simulink model "Horticulture_Simulation_2"  (R2025a)
settings: Solver=ode45  StartTime=0.0  StopTime=100000  RelTol=1e-3
libraries: simulink x9, slpidlib x2
settings Model: Creator=VICTUS  LastModifiedBy=VICTUS

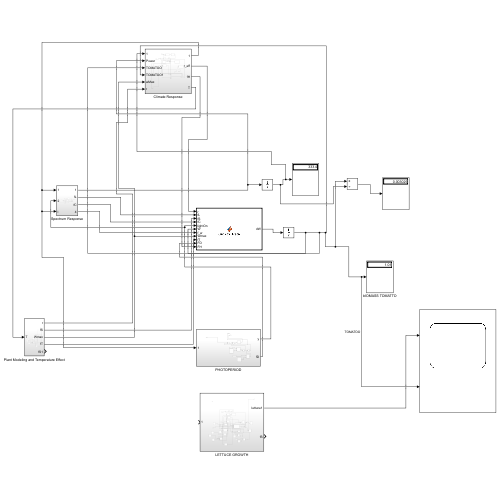
[thumbnail: Simulink's stored preview of the top-level diagram]
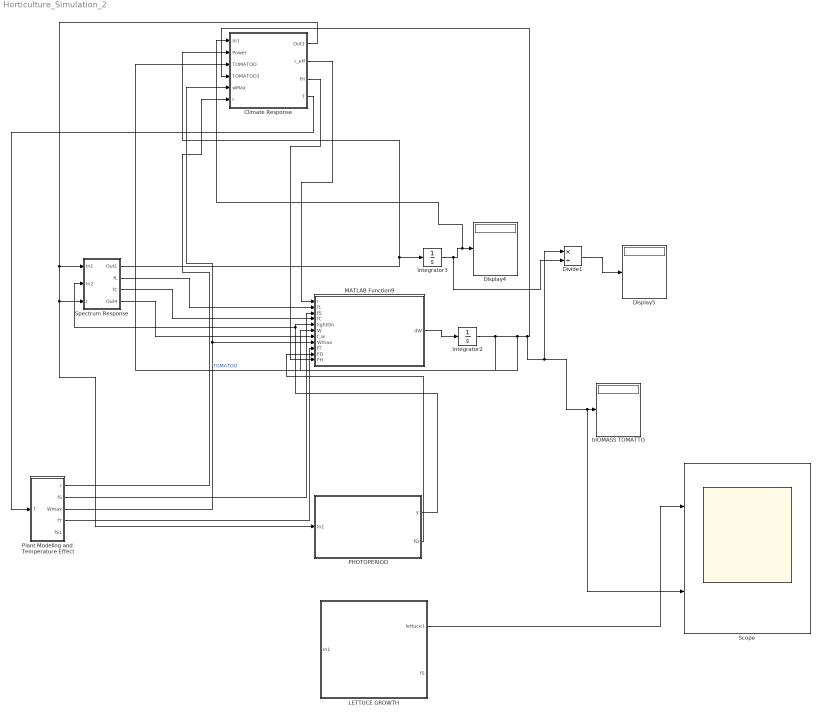
== system Horticulture_Simulation_2 ==
  Climate Response : Subsystem
  Display4 : Display
  Display5 : Display
  Divide1 : Product  Inputs=*/
  Integrator2 : Integrator  InitialCondition=1
  Integrator3 : Integrator
  LETTUCE GROWTH : Subsystem
  MATLAB Function9 : MATLAB Function  TreatAsAtomicUnit=on
  PHOTOPERIOD : Subsystem
  Plant Modeling and Temperature Effect : Subsystem
  Scope : Scope  NumInputPorts=2
      settings: ActiveDisplayYMinimum=0.99710090280302532  ActiveDisplayYMaximum=1.0260918747727719
  Spectrum Response : Subsystem
  bIOMASS TOMATTO : Display
  wires:
  Integrator2/1 -> Climate Response/3(TOMATOO), Climate Response/4(TOMATOO1), Divide1/1, Scope/2, bIOMASS TOMATTO/1, MATLAB Function9/6(W)  "TOMATOO"
  Divide1/1 -> Display5/1
  MATLAB Function9/1(dW) -> Integrator2/1
  Integrator3/1 -> Divide1/2, Climate Response/1(In1), Display4/1
  PHOTOPERIOD/1(y) -> Spectrum Response/2(In2), MATLAB Function9/5(lightOn)
  PHOTOPERIOD/2(fD) -> MATLAB Function9/10(FD)
  Plant Modeling and Temperature Effect/3(Wmax) -> Climate Response/5(wMax), MATLAB Function9/8(Wmax)
  Plant Modeling and Temperature Effect/2(fS) -> MATLAB Function9/3(fS)
  Plant Modeling and Temperature Effect/4(fT) -> MATLAB Function9/9(fT)
  Climate Response/1(Out1) -> PHOTOPERIOD/1(In1), Spectrum Response/3(I), Spectrum Response/1(In1)
  Plant Modeling and Temperature Effect/1(r) -> Climate Response/6(r)
  Climate Response/2(r_eff) -> MATLAB Function9/1(r)
  Climate Response/3(fH) -> MATLAB Function9/11(FH)
  Climate Response/4(T) -> Plant Modeling and Temperature Effect/1(T)
  Spectrum Response/1(Out1) -> Climate Response/2(Power), Integrator3/1
  Spectrum Response/2(fL) -> MATLAB Function9/2(fL)
  Spectrum Response/3(fC) -> MATLAB Function9/4(fC)
  Spectrum Response/4(Out4) -> MATLAB Function9/7(f_w)
  LETTUCE GROWTH/1(lettuce1) -> Scope/1

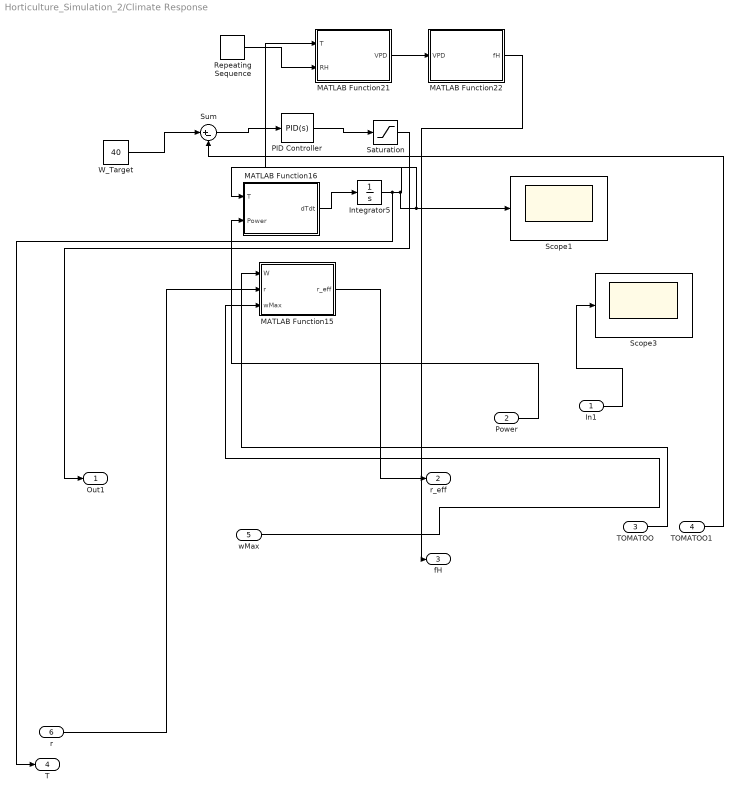
== system Horticulture_Simulation_2/Climate Response ==
  In1 : Inport
  Power : Inport  Port=2
  TOMATOO : Inport  Port=3
  TOMATOO1 : Inport  Port=4
  wMax : Inport  Port=5
  r : Inport  Port=6
  Integrator5 : Integrator  InitialCondition=22
  MATLAB Function15 : MATLAB Function  TreatAsAtomicUnit=on
  MATLAB Function16 : MATLAB Function  TreatAsAtomicUnit=on
  MATLAB Function21 : MATLAB Function  TreatAsAtomicUnit=on
  MATLAB Function22 : MATLAB Function  TreatAsAtomicUnit=on
  PID Controller : slpidlib/PID Controller  Controller=PID  Form=Parallel  TimeDomain=Continuous-time  UseExternalTs=off  SampleTime=-1  IntegratorMethod=Forward Euler  FilterMethod=Forward Euler  ControllerParametersSource=internal  P=0.5  I=0.01  UseKiTs=off  D=0  UseExternalDerivativeSource=off  N=100  UseFilter=on  TunerSelectOption=Transfer Function Based (PID Tuner App)  InitialConditionSource=internal  InitialConditionForIntegrator=0  InitialConditionForFilter=0  DifferentiatorICPrevScaledInput=0  ExternalReset=none  TrackingMode=off  Kt=1  LimitOutput=off  SatLimitsSource=internal  UpperSaturationLimit=inf  LowerSaturationLimit=-inf  LinearizeAsGain=on  AntiWindupMode=none  Kb=1  LimitIntegrator=off  UpperIntegratorSaturationLimit=inf  LowerIntegratorSaturationLimit=-inf  POutMin=[]  POutMax=[]  IOutMin=[]  IOutMax=[]  DOutMin=[]  DOutMax=[]  NOutMin=[]  NOutMax=[]  SumOutMin=[]  SumOutMax=[]  SaturationOutMin=[]  SaturationOutMax=[]  PParamMin=[]  PParamMax=[]  IParamMin=[]  IParamMax=[]  DParamMin=[]  DParamMax=[]  NParamMin=[]  NParamMax=[]  KbParamMin=[]  KbParamMax=[]  KtParamMin=[]  KtParamMax=[]  KbOutMin=[]  KbOutMax=[]  KtOutMin=[]  KtOutMax=[]  IntegratorOutMin=[]  IntegratorOutMax=[]  FilterOutMin=[]  FilterOutMax=[]  SumI1OutMin=[]  SumI1OutMax=[]  SumI2OutMin=[]  SumI2OutMax=[]  SumI3OutMin=[]  SumI3OutMax=[]  SumI4OutMin=[]  SumI4OutMax=[]  SumDOutMin=[]  SumDOutMax=[]  DifferentiatorOutMin=[]  DifferentiatorOutMax=[]  FilterDiffOutCoefMin=[]  FilterDiffOutCoefMax=[]  ReciprocalOutMin=[]  ReciprocalOutMax=[]  SumDenOutMin=[]  SumDenOutMax=[]  SumNumOutMin=[]  SumNumOutMax=[]  DivideOutMin=[]  DivideOutMax=[]  UdiffTsProdOutMin=[]  UdiffTsProdOutMax=[]  NTsProdOutMin=[]  NTsProdOutMax=[]  UintegralTsProdOutMin=[]  UintegralTsProdOutMax=[]  UngainTsProdOutMin=[]  UngainTsProdOutMax=[]  ClampingZeroOutDataTypeStr=Inherit: Inherit via back propagation  ClampingZeroOutMin=[]  ClampingZeroOutMax=[]  FilterDenConstantOutDataTypeStr=Inherit: Inherit via back propagation  FilterDenConstantOutMin=[]  FilterDenConstantOutMax=[]  PCopyOutDataTypeStr=Inherit: Inherit via back propagation  PCopyOutMin=[]  PCopyOutMax=[]  NCopyOutDataTypeStr=Inherit: Inherit via back propagation  NCopyOutMin=[]  NCopyOutMax=[]  IntegratorContinuousStateAttributes=''  IntegratorStateMustResolveToSignalObject=off  IntegratorRTWStateStorageClass=Auto  FilterContinuousStateAttributes=''  FilterStateMustResolveToSignalObject=off  FilterRTWStateStorageClass=Auto  ParallelPVariant=InternalParameters  IdealPVariant=Disabled  IVariant=InternalParameters  DVariant=InternalParameters  IntegratorVariant=Continuous  SatVariant=Disabled  AWVariant=Passthrough  PCopyVariant=Disabled  TRVariant=Disabled  FdbkBlocksVariant=Forward  IdealPFdbkVariant=Disabled  SatFdbkVariant=Disabled  DerivativeFilterVariant=ContFilter  NVariant=InternalParameters  NCopyVariant=Disabled  FilterICVariant=InternalICsFilter  IntegratorICVariant=InternalICs  ExternalResetVariant=Disabled  TRSumVariant=Passthrough  SumFdbkVariant=Disabled  SumVariant=Sum_PID  TsampFilterVariant=InternalTs  TsampNgainVariant=Passthrough  TsampIntegralVariant=Disabled_SignalSpec  ExternalSaturationOutDataTypeStr=Inherit: Same as second input  DerivativeSourceVariant=ErrorSignal  PreIntVariant=InternalPreInt
  Repeating Sequence : simulink/Sources/Repeating Sequence  rep_seq_t=[0 16 24]  rep_seq_y=[60 80 60]
  Saturation : Saturate
  Scope1 : Scope
      settings: ActiveDisplayYMinimum=22.738000496839618  ActiveDisplayYMaximum=28.32565714151929
  Scope3 : Scope
      settings: ActiveDisplayYMinimum=-0.063605341937586823  ActiveDisplayYMaximum=0.39000361099138614  DataLoggingVariableName=ScopeData3
  Sum : Sum  Inputs=|+-
  W_Target : Constant  Value=40
  Out1 : Outport
  r_eff : Outport  Port=2
  fH : Outport  Port=3
  T : Outport  Port=4
  wires:
  TOMATOO1/1 -> Sum/2
  PID Controller/1 -> Saturation/1
  Sum/1 -> PID Controller/1
  Repeating Sequence/1 -> MATLAB Function21/2(RH)
  Integrator5/1 -> T/1, MATLAB Function21/1(T), Scope1/1, MATLAB Function16/1(T)
  W_Target/1 -> Sum/1
  MATLAB Function16/1(dTdt) -> Integrator5/1
  MATLAB Function21/1(VPD) -> MATLAB Function22/1(VPD)
  Saturation/1 -> Out1/1
  MATLAB Function15/1(r_eff) -> r_eff/1
  Power/1 -> MATLAB Function16/2(Power)
  wMax/1 -> MATLAB Function15/3(wMax)
  TOMATOO/1 -> MATLAB Function15/1(W)
  In1/1 -> Scope3/1
  r/1 -> MATLAB Function15/2(r)
  MATLAB Function22/1(fH) -> fH/1

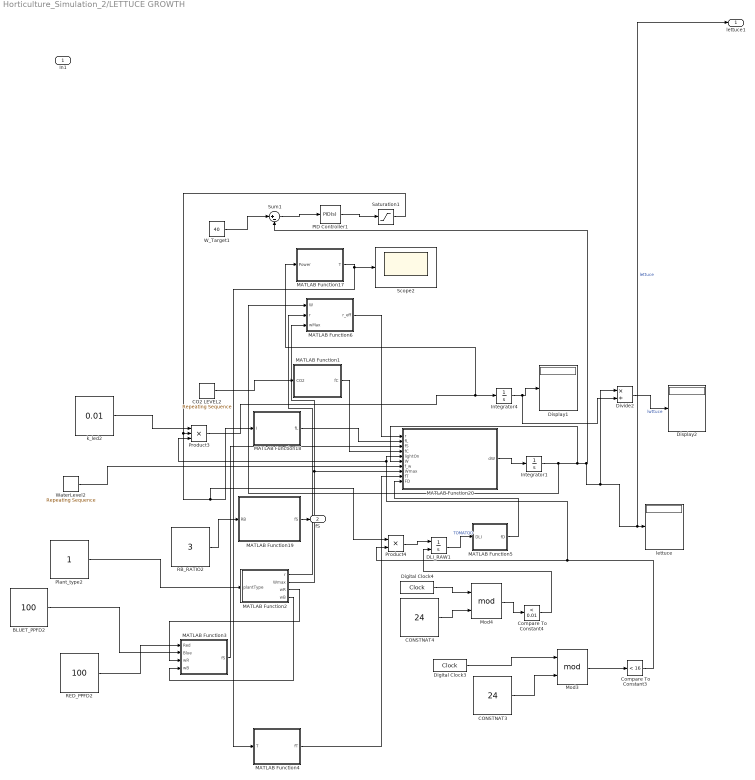
== system Horticulture_Simulation_2/LETTUCE GROWTH ==
  In1 : Inport
  BLUET_PPFD2 : Constant  Value=100
  CO2 LEVEL2 : simulink/Sources/Repeating Sequence  rep_seq_t=[0 16 24]  rep_seq_y=[800 400 800]
  CONSTNAT3 : Constant  Value=24
  CONSTNAT4 : Constant  Value=24
  Compare To Constant3 : simulink/Logic and Bit Operations/Compare To Constant  relop=<  const=16  OutDataTypeStr=boolean
  Compare To Constant4 : simulink/Logic and Bit Operations/Compare To Constant  relop=<  const=0.01  OutDataTypeStr=boolean
  DLI_RAW1 : Integrator  ExternalReset=either
  Digital Clock3 : DigitalClock
  Digital Clock4 : DigitalClock
  Display1 : Display
  Display2 : Display
  Divide2 : Product  Inputs=*/
  Integrator1 : Integrator  InitialCondition=1
  Integrator4 : Integrator
  MATLAB Function1 : MATLAB Function  TreatAsAtomicUnit=on
  MATLAB Function17 : MATLAB Function  TreatAsAtomicUnit=on
  MATLAB Function18 : MATLAB Function  TreatAsAtomicUnit=on
  MATLAB Function19 : MATLAB Function  TreatAsAtomicUnit=on
  MATLAB Function2 : MATLAB Function  TreatAsAtomicUnit=on
  MATLAB Function20 : MATLAB Function  TreatAsAtomicUnit=on
  MATLAB Function3 : MATLAB Function  TreatAsAtomicUnit=on
  MATLAB Function4 : MATLAB Function  TreatAsAtomicUnit=on
  MATLAB Function5 : MATLAB Function  TreatAsAtomicUnit=on
  MATLAB Function6 : MATLAB Function  TreatAsAtomicUnit=on
  Mod3 : Math  Operator=mod
  Mod4 : Math  Operator=mod
  PID Controller1 : slpidlib/PID Controller  Controller=PID  Form=Parallel  TimeDomain=Continuous-time  UseExternalTs=off  SampleTime=-1  IntegratorMethod=Forward Euler  FilterMethod=Forward Euler  ControllerParametersSource=internal  P=0.5  I=0.01  UseKiTs=off  D=0  UseExternalDerivativeSource=off  N=100  UseFilter=on  TunerSelectOption=Transfer Function Based (PID Tuner App)  InitialConditionSource=internal  InitialConditionForIntegrator=0  InitialConditionForFilter=0  DifferentiatorICPrevScaledInput=0  ExternalReset=none  TrackingMode=off  Kt=1  LimitOutput=off  SatLimitsSource=internal  UpperSaturationLimit=inf  LowerSaturationLimit=-inf  LinearizeAsGain=on  AntiWindupMode=none  Kb=1  LimitIntegrator=off  UpperIntegratorSaturationLimit=inf  LowerIntegratorSaturationLimit=-inf  POutMin=[]  POutMax=[]  IOutMin=[]  IOutMax=[]  DOutMin=[]  DOutMax=[]  NOutMin=[]  NOutMax=[]  SumOutMin=[]  SumOutMax=[]  SaturationOutMin=[]  SaturationOutMax=[]  PParamMin=[]  PParamMax=[]  IParamMin=[]  IParamMax=[]  DParamMin=[]  DParamMax=[]  NParamMin=[]  NParamMax=[]  KbParamMin=[]  KbParamMax=[]  KtParamMin=[]  KtParamMax=[]  KbOutMin=[]  KbOutMax=[]  KtOutMin=[]  KtOutMax=[]  IntegratorOutMin=[]  IntegratorOutMax=[]  FilterOutMin=[]  FilterOutMax=[]  SumI1OutMin=[]  SumI1OutMax=[]  SumI2OutMin=[]  SumI2OutMax=[]  SumI3OutMin=[]  SumI3OutMax=[]  SumI4OutMin=[]  SumI4OutMax=[]  SumDOutMin=[]  SumDOutMax=[]  DifferentiatorOutMin=[]  DifferentiatorOutMax=[]  FilterDiffOutCoefMin=[]  FilterDiffOutCoefMax=[]  ReciprocalOutMin=[]  ReciprocalOutMax=[]  SumDenOutMin=[]  SumDenOutMax=[]  SumNumOutMin=[]  SumNumOutMax=[]  DivideOutMin=[]  DivideOutMax=[]  UdiffTsProdOutMin=[]  UdiffTsProdOutMax=[]  NTsProdOutMin=[]  NTsProdOutMax=[]  UintegralTsProdOutMin=[]  UintegralTsProdOutMax=[]  UngainTsProdOutMin=[]  UngainTsProdOutMax=[]  ClampingZeroOutDataTypeStr=Inherit: Inherit via back propagation  ClampingZeroOutMin=[]  ClampingZeroOutMax=[]  FilterDenConstantOutDataTypeStr=Inherit: Inherit via back propagation  FilterDenConstantOutMin=[]  FilterDenConstantOutMax=[]  PCopyOutDataTypeStr=Inherit: Inherit via back propagation  PCopyOutMin=[]  PCopyOutMax=[]  NCopyOutDataTypeStr=Inherit: Inherit via back propagation  NCopyOutMin=[]  NCopyOutMax=[]  IntegratorContinuousStateAttributes=''  IntegratorStateMustResolveToSignalObject=off  IntegratorRTWStateStorageClass=Auto  FilterContinuousStateAttributes=''  FilterStateMustResolveToSignalObject=off  FilterRTWStateStorageClass=Auto  ParallelPVariant=InternalParameters  IdealPVariant=Disabled  IVariant=InternalParameters  DVariant=InternalParameters  IntegratorVariant=Continuous  SatVariant=Disabled  AWVariant=Passthrough  PCopyVariant=Disabled  TRVariant=Disabled  FdbkBlocksVariant=Forward  IdealPFdbkVariant=Disabled  SatFdbkVariant=Disabled  DerivativeFilterVariant=ContFilter  NVariant=InternalParameters  NCopyVariant=Disabled  FilterICVariant=InternalICsFilter  IntegratorICVariant=InternalICs  ExternalResetVariant=Disabled  TRSumVariant=Passthrough  SumFdbkVariant=Disabled  SumVariant=Sum_PID  TsampFilterVariant=InternalTs  TsampNgainVariant=Passthrough  TsampIntegralVariant=Disabled_SignalSpec  ExternalSaturationOutDataTypeStr=Inherit: Same as second input  DerivativeSourceVariant=ErrorSignal  PreIntVariant=InternalPreInt
  Plant_type2 : Constant
  Product3 : Product  Inputs=3
  Product4 : Product
  RB_RATIO2 : Constant  Value=3
  RED_PPFD2 : Constant  Value=100
  Saturation1 : Saturate
  Scope2 : Scope
      settings: ActiveDisplayYMinimum=17  ActiveDisplayYMaximum=67  DataLoggingVariableName=ScopeData2
  Sum1 : Sum  Inputs=|+-
  W_Target1 : Constant  Value=40
  WaterLevel2 : simulink/Sources/Repeating Sequence  rep_seq_t=[0 12 24]  rep_seq_y=[1 0.6 1]
  k_led2 : Constant  Value=0.01
  lettuce : Display
  lettuce1 : Outport
  fS : Outport  Port=2
  wires:
  MATLAB Function5/1(fD) -> MATLAB Function20/10(FD)
  CO2 LEVEL2/1 -> MATLAB Function1/1(CO2)
  MATLAB Function20/1(dW) -> Integrator1/1
  MATLAB Function2/1(r) -> MATLAB Function6/2(r)
  RB_RATIO2/1 -> MATLAB Function19/1(RB)
  Mod4/1 -> Compare To Constant4/1
  RED_PPFD2/1 -> MATLAB Function3/1(Red)
  Integrator4/1 -> Divide2/2, Display1/1
  Product4/1 -> DLI_RAW1/1
  Product3/1 -> MATLAB Function17/1(Power), Integrator4/1
  MATLAB Function17/1(T) -> MATLAB Function4/1(T), Scope2/1
  Divide2/1 -> Display2/1  "lwttuce"
  Digital Clock4/1 -> Mod4/1
  MATLAB Function2/2(Wmax) -> MATLAB Function6/3(wMax), MATLAB Function20/8(Wmax)
  Mod3/1 -> Compare To Constant3/1
  Compare To Constant3/1 -> Product4/2, Product3/3, MATLAB Function20/5(lightOn)
  MATLAB Function4/1(fT) -> MATLAB Function20/9(fT)
  MATLAB Function3/1(fS) -> MATLAB Function20/3(fS)
  MATLAB Function2/4(wB) -> MATLAB Function3/4(wB)
  Integrator1/1 -> Sum1/2, Divide2/1, lettuce1/1, lettuce/1, MATLAB Function20/6(W), MATLAB Function6/1(W)  "lettuce"
  k_led2/1 -> Product3/1
  PID Controller1/1 -> Saturation1/1
  MATLAB Function2/3(wR) -> MATLAB Function3/3(wR)
  BLUET_PPFD2/1 -> MATLAB Function3/2(Blue)
  CONSTNAT4/1 -> Mod4/2
  MATLAB Function1/1(fC) -> MATLAB Function20/4(fC)
  Saturation1/1 -> Product4/1, MATLAB Function18/1(I), Product3/2
  Plant_type2/1 -> MATLAB Function2/1(plantType)
  WaterLevel2/1 -> MATLAB Function20/7(f_w)
  Sum1/1 -> PID Controller1/1
  Digital Clock3/1 -> Mod3/1
  MATLAB Function18/1(fL) -> MATLAB Function20/2(fL)
  MATLAB Function6/1(r_eff) -> MATLAB Function20/1(r)
  DLI_RAW1/1 -> MATLAB Function5/1(DLI)  "TOMATOO"
  W_Target1/1 -> Sum1/1
  CONSTNAT3/1 -> Mod3/2
  MATLAB Function19/1(fS) -> fS/1
  Compare To Constant4/1 -> DLI_RAW1/2

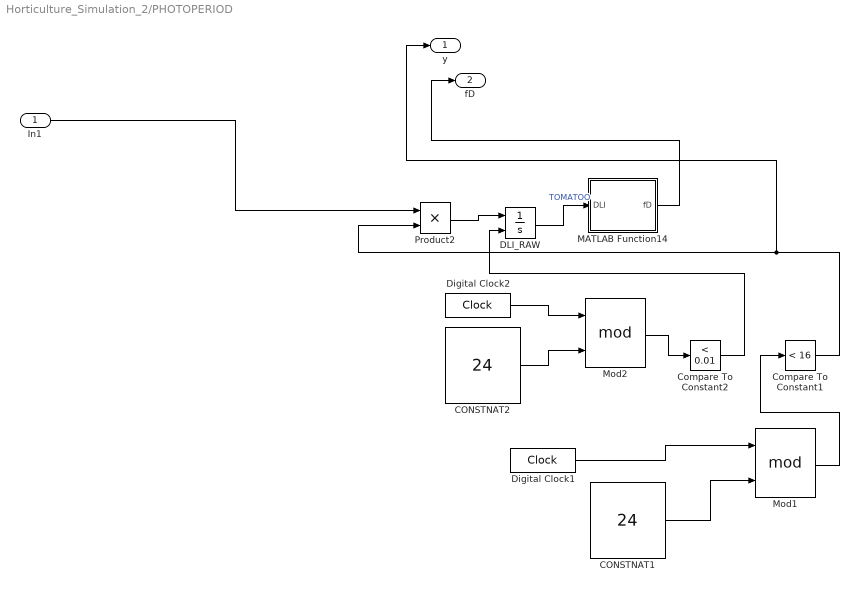
== system Horticulture_Simulation_2/PHOTOPERIOD ==
  In1 : Inport
  CONSTNAT1 : Constant  Value=24
  CONSTNAT2 : Constant  Value=24
  Compare To Constant1 : simulink/Logic and Bit Operations/Compare To Constant  relop=<  const=16  OutDataTypeStr=boolean
  Compare To Constant2 : simulink/Logic and Bit Operations/Compare To Constant  relop=<  const=0.01  OutDataTypeStr=boolean
  DLI_RAW : Integrator  ExternalReset=either
  Digital Clock1 : DigitalClock
  Digital Clock2 : DigitalClock
  MATLAB Function14 : MATLAB Function  TreatAsAtomicUnit=on
  Mod1 : Math  Operator=mod
  Mod2 : Math  Operator=mod
  Product2 : Product
  y : Outport
  fD : Outport  Port=2
  wires:
  Digital Clock2/1 -> Mod2/1
  Compare To Constant1/1 -> y/1, Product2/2
  Mod1/1 -> Compare To Constant1/1
  CONSTNAT2/1 -> Mod2/2
  Product2/1 -> DLI_RAW/1
  Digital Clock1/1 -> Mod1/1
  CONSTNAT1/1 -> Mod1/2
  Compare To Constant2/1 -> DLI_RAW/2
  Mod2/1 -> Compare To Constant2/1
  DLI_RAW/1 -> MATLAB Function14/1(DLI)  "TOMATOO"
  In1/1 -> Product2/1
  MATLAB Function14/1(fD) -> fD/1

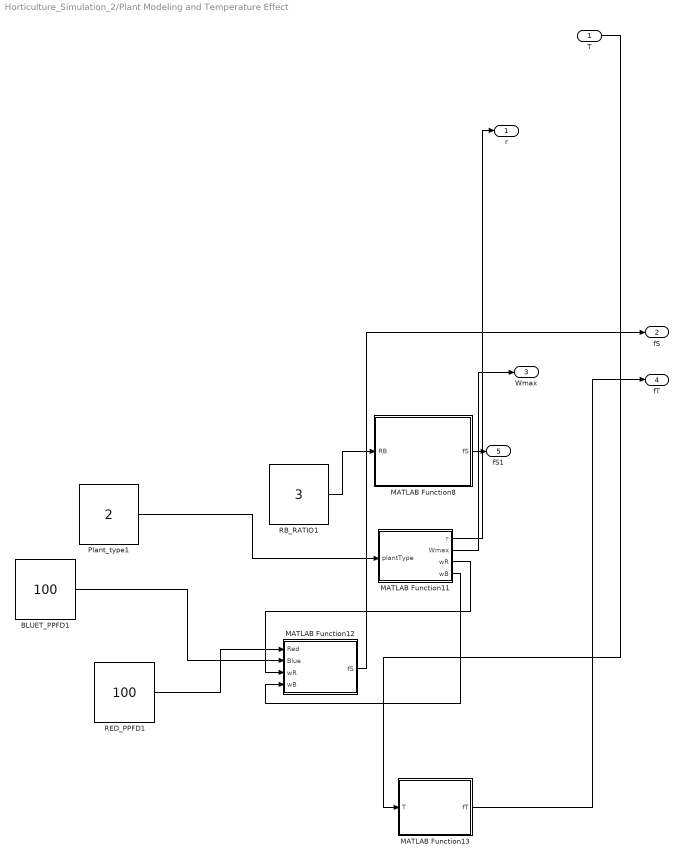
== system Horticulture_Simulation_2/Plant Modeling and Temperature Effect ==
  T : Inport
  BLUET_PPFD1 : Constant  Value=100
  MATLAB Function11 : MATLAB Function  TreatAsAtomicUnit=on
  MATLAB Function12 : MATLAB Function  TreatAsAtomicUnit=on
  MATLAB Function13 : MATLAB Function  TreatAsAtomicUnit=on
  MATLAB Function8 : MATLAB Function  TreatAsAtomicUnit=on
  Plant_type1 : Constant  Value=2
  RB_RATIO1 : Constant  Value=3
  RED_PPFD1 : Constant  Value=100
  r : Outport
  fS : Outport  Port=2
  Wmax : Outport  Port=3
  fT : Outport  Port=4
  fS1 : Outport  Port=5
  wires:
  RED_PPFD1/1 -> MATLAB Function12/1(Red)
  MATLAB Function13/1(fT) -> fT/1
  MATLAB Function11/2(Wmax) -> Wmax/1
  MATLAB Function11/3(wR) -> MATLAB Function12/3(wR)
  BLUET_PPFD1/1 -> MATLAB Function12/2(Blue)
  MATLAB Function11/4(wB) -> MATLAB Function12/4(wB)
  RB_RATIO1/1 -> MATLAB Function8/1(RB)
  Plant_type1/1 -> MATLAB Function11/1(plantType)
  MATLAB Function12/1(fS) -> fS/1
  MATLAB Function11/1(r) -> r/1
  MATLAB Function8/1(fS) -> fS1/1
  T/1 -> MATLAB Function13/1(T)

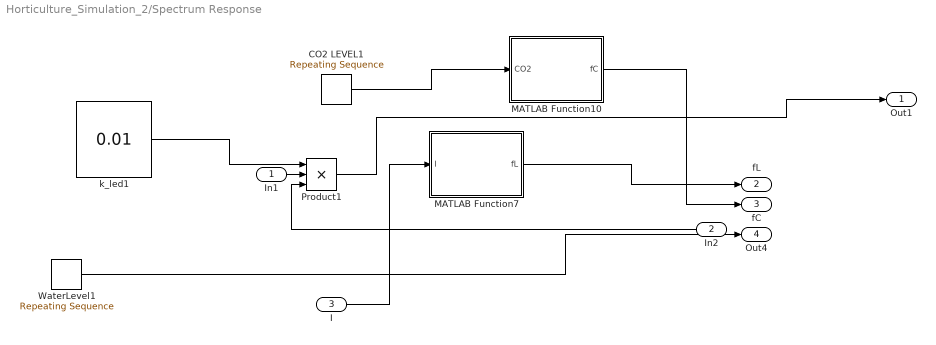
== system Horticulture_Simulation_2/Spectrum Response ==
  In1 : Inport
  In2 : Inport  Port=2
  I : Inport  Port=3
  CO2 LEVEL1 : simulink/Sources/Repeating Sequence  rep_seq_t=[0 16 24]  rep_seq_y=[800 400 800]
  MATLAB Function10 : MATLAB Function  TreatAsAtomicUnit=on
  MATLAB Function7 : MATLAB Function  TreatAsAtomicUnit=on
  Product1 : Product  Inputs=3
  WaterLevel1 : simulink/Sources/Repeating Sequence  rep_seq_t=[0 12 24]  rep_seq_y=[1 0.6 1]
  k_led1 : Constant  Value=0.01
  Out1 : Outport
  fL : Outport  Port=2
  fC : Outport  Port=3
  Out4 : Outport  Port=4
  wires:
  k_led1/1 -> Product1/1
  MATLAB Function7/1(fL) -> fL/1
  WaterLevel1/1 -> Out4/1
  In2/1 -> Product1/3
  CO2 LEVEL1/1 -> MATLAB Function10/1(CO2)
  In1/1 -> Product1/2
  Product1/1 -> Out1/1
  I/1 -> MATLAB Function7/1(I)
  MATLAB Function10/1(fC) -> fC/1

== matlab function Horticulture_Simulation_2/Plant Modeling and Temperature Effect/MATLAB Function13 ==
  data: T input; fT output
function fT = Temp_Response(T)

Topt = 22;   % optimal temperature
sigma = 7;   % tolerance

fT = exp(-((T - Topt)^2) / (2*sigma^2));

end

== matlab function Horticulture_Simulation_2/Spectrum Response/MATLAB Function7 ==
  data: I input; fL output
function fL = Light_Response(I)
Isat = 300; % saturation point
fL = I / (I + Isat);
end

== matlab function Horticulture_Simulation_2/Plant Modeling and Temperature Effect/MATLAB Function8 ==
  data: RB input; fS output
function fS = Spectrum_Response(RB)
RBopt = 3;
ks = 0.1;

fS = 1 + ks*(RB - RBopt);
fS = min(max(fS,0),1.2);
end

== matlab function Horticulture_Simulation_2/MATLAB Function9 ==
  data: r input; fL input; dW output; fS input; fC input; lightOn input; W input; f_w input; Wmax input; fT input; FD input; FH input
function dW = Growth_Rate(r,fL, fS, fC, lightOn, W,f_w,Wmax,fT,FD,FH)



dW = r * fL * fS * fC * lightOn * (1 - W/Wmax)*f_w*fT*FD*FH;
end

== matlab function Horticulture_Simulation_2/PHOTOPERIOD/MATLAB Function14 ==
  data: DLI input; fD output
function fD = DLI_Response(DLI)

DLI_sat = 20;   % normalized
fD = DLI / (DLI + DLI_sat);

end

== matlab function Horticulture_Simulation_2/Climate Response/MATLAB Function15 ==
  data: W input; r_eff output; r input; wMax input
function r_eff = Stage_Modifier(W, r,wMax)

if W < 0.2*wMax       % seedling
    r_eff = 0.4*r;
elseif W < 0.7*wMax   % vegetative
    r_eff = r;
else                % mature
    r_eff = 0.3*r;
end

end

== matlab function Horticulture_Simulation_2/Climate Response/MATLAB Function16 ==
  data: T input; Power input; dTdt output
function dTdt = Thermal_Dynamics(T, Power)

Tamb = 22;
k_heat = 250;     % heating strength
k_cool = 0.2;     % cooling strength

dTdt = k_heat*Power - k_cool*(T - Tamb);

end

== matlab function Horticulture_Simulation_2/LETTUCE GROWTH/MATLAB Function4 ==
  data: T input; fT output
function fT = Temp_Response(T)

Topt = 22;   % optimal temperature
sigma = 7;   % tolerance

fT = exp(-((T - Topt)^2) / (2*sigma^2));

end

== matlab function Horticulture_Simulation_2/LETTUCE GROWTH/MATLAB Function5 ==
  data: DLI input; fD output
function fD = DLI_Response(DLI)

DLI_sat = 20;   % normalized
fD = DLI / (DLI + DLI_sat);

end

== matlab function Horticulture_Simulation_2/LETTUCE GROWTH/MATLAB Function1 ==
  data: CO2 input; fC output
function fC = CO2_Response(CO2)
CO2sat = 800;   % ppm
fC = CO2 / (CO2 + CO2sat);
end

== matlab function Horticulture_Simulation_2/LETTUCE GROWTH/MATLAB Function6 ==
  data: W input; r_eff output; r input; wMax input
function r_eff = Stage_Modifier(W, r,wMax)

if W < 0.2*wMax       % seedling
    r_eff = 0.4*r;
elseif W < 0.7*wMax   % vegetative
    r_eff = r;
else                % mature
    r_eff = 0.3*r;
end

end

== matlab function Horticulture_Simulation_2/Climate Response/MATLAB Function21 ==
  data: T input; RH input; VPD output
function VPD = VPD_Model(T, RH)
% T in °C, RH in %

es = 0.6108 * exp((17.27*T)/(T+237.3)); % saturation vapor pressure (kPa)
ea = es * (RH/100);

VPD = es - ea;  % kPa
end

== matlab function Horticulture_Simulation_2/Climate Response/MATLAB Function22 ==
  data: VPD input; fH output
function fH = VPD_Response(VPD)

VPD_opt = 1.2;   % kPa (greenhouse typical)
sigma = 0.5;

fH = exp(-((VPD - VPD_opt)^2)/(2*sigma^2));
end

== matlab function Horticulture_Simulation_2/LETTUCE GROWTH/MATLAB Function17 ==
  data: Power input; T output
function T = LED_Heat_Model(Power)

Tamb = 22;       % ambient
k_heat = 2;      % °C per kW

T = Tamb + k_heat * Power;

end

== matlab function Horticulture_Simulation_2/LETTUCE GROWTH/MATLAB Function18 ==
  data: I input; fL output
function fL = Light_Response(I)
Isat = 300; % saturation point
fL = I / (I + Isat);
end

== matlab function Horticulture_Simulation_2/LETTUCE GROWTH/MATLAB Function19 ==
  data: RB input; fS output
function fS = Spectrum_Response(RB)
RBopt = 3;
ks = 0.1;

fS = 1 + ks*(RB - RBopt);
fS = min(max(fS,0),1.2);
end

== matlab function Horticulture_Simulation_2/LETTUCE GROWTH/MATLAB Function2 ==
  data: plantType input; r output; Wmax output; wR output; wB output
function [r, Wmax, wR, wB] = Plant_Params(plantType)

if plantType == 1      % Lettuce
    r    = 0.04;
    Wmax = 50;
    wR   = 0.6;
    wB   = 0.4;
else                  % Tomato
    r    = 0.025;
    Wmax = 200;
    wR   = 0.8;
    wB   = 0.2;
end

== matlab function Horticulture_Simulation_2/LETTUCE GROWTH/MATLAB Function20 ==
  data: r input; fL input; dW output; fS input; fC input; lightOn input; W input; f_w input; Wmax input; fT input; FD input
function dW = Growth_Rate(r,fL, fS, fC, lightOn, W,f_w,Wmax,fT,FD)



dW = r * fL * fS * fC * lightOn * (1 - W/Wmax)*f_w*fT*FD;
end

== matlab function Horticulture_Simulation_2/LETTUCE GROWTH/MATLAB Function3 ==
  data: Red input; fS output; Blue input; wR input; wB input
function fS = Spectrum_Model(Red, Blue, wR, wB)

% Normalize light
Red_n  = Red  / (Red  + 200);
Blue_n = Blue / (Blue + 200);

% Weighted response
fS = wR * Red_n + wB * Blue_n;

% Safety clamp
fS = min(max(fS, 0), 1);

end

== matlab function Horticulture_Simulation_2/Spectrum Response/MATLAB Function10 ==
  data: CO2 input; fC output
function fC = CO2_Response(CO2)
CO2sat = 800;   % ppm
fC = CO2 / (CO2 + CO2sat);
end

== matlab function Horticulture_Simulation_2/Plant Modeling and Temperature Effect/MATLAB Function11 ==
  data: plantType input; r output; Wmax output; wR output; wB output
function [r, Wmax, wR, wB] = Plant_Params(plantType)

if plantType == 1      % Lettuce
    r    = 0.04;
    Wmax = 50;
    wR   = 0.6;
    wB   = 0.4;
else                  % Tomato
    r    = 0.025;
    Wmax = 200;
    wR   = 0.8;
    wB   = 0.2;
end

== matlab function Horticulture_Simulation_2/Plant Modeling and Temperature Effect/MATLAB Function12 ==
  data: Red input; fS output; Blue input; wR input; wB input
function fS = Spectrum_Model(Red, Blue, wR, wB)

% Normalize light
Red_n  = Red  / (Red  + 200);
Blue_n = Blue / (Blue + 200);

% Weighted response
fS = wR * Red_n + wB * Blue_n;

% Safety clamp
fS = min(max(fS, 0), 1);

end
